simulink model "FK"  (R2024b)
settings: Solver=FixedStepDiscrete  StartTime=0.0  StopTime=Inf  FixedStep=0.001  RelTol=1e-3
model workspace (MAT data in the model file):
  robot : robotics.RigidBodyTree (value not decoded)
values from neighbouring files (symbols this model uses):
  lambda_l_list = [lambda_l_list,se3ToVec(logm(getTransform(robot,q,"l_tcp","l_6")))]    [getDualArmLambdaList.m]
  lambda_rl_list = [lambda_rl_list,se3ToVec(logm(getTransform(robot,q,"l_tcp","l_6")))]    [getDualArmLambdaList.m]
undefined symbols (not defined in the file or in its folder): lambda_r_list
settings Model: Creator=sung  LastModifiedBy=sung
settings HardwareCC: ProdBitPerLong=64  ProdHWDeviceType=Intel->x86-64 (Linux 64)
settings RTWCC: GenCodeOnly=on  Toolchain=CMake

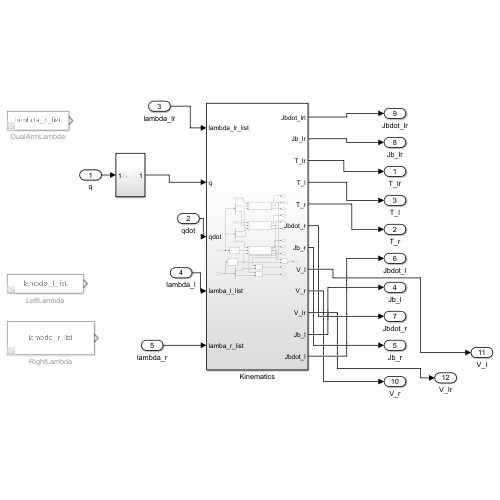
[thumbnail: Simulink's stored preview of the top-level diagram]
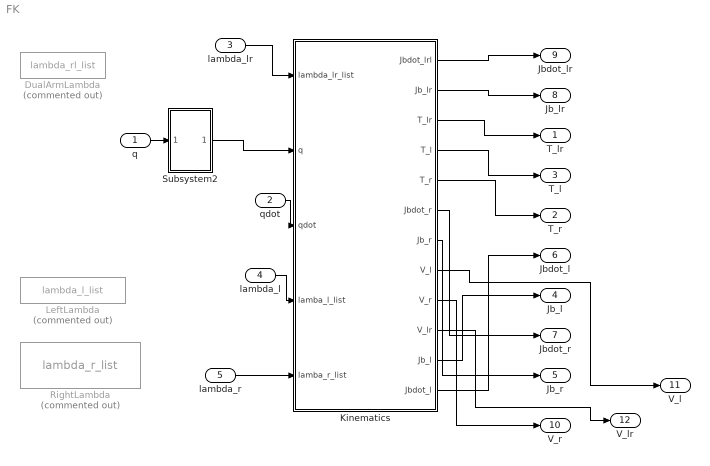
== system FK ==
  q : Inport  PortDimensions=12
  qdot : Inport  Port=2  PortDimensions=12
  lambda_lr : Inport  Port=3  PortDimensions=[6,13]
  lambda_l : Inport  Port=4  PortDimensions=[6,7]
  lambda_r : Inport  Port=5  PortDimensions=[6,7]
  DualArmLambda : Constant  Commented=on  Value=lambda_rl_list
  Kinematics : Subsystem
  LeftLambda : Constant  Commented=on  Value=lambda_l_list
  RightLambda : Constant  Commented=on  Value=lambda_r_list
  Subsystem2 : Subsystem
  T_lr : Outport
  T_r : Outport  Port=2
  T_l : Outport  Port=3
  Jb_l : Outport  Port=4
  Jb_r : Outport  Port=5
  Jbdot_l : Outport  Port=6
  Jbdot_r : Outport  Port=7
  Jb_lr : Outport  Port=8
  Jbdot_lr : Outport  Port=9
  V_r : Outport  Port=10
  V_l : Outport  Port=11
  V_lr : Outport  Port=12
  wires:
  Kinematics/4(T_l) -> T_l/1
  Kinematics/5(T_r) -> T_r/1
  Kinematics/3(T_lr) -> T_lr/1
  Kinematics/2(Jb_lr) -> Jb_lr/1
  Kinematics/1(Jbdot_lrl) -> Jbdot_lr/1
  q/1 -> Subsystem2/1(In1)
  qdot/1 -> Kinematics/3(qdot)
  lambda_lr/1 -> Kinematics/1(lambda_lr_list)
  lambda_l/1 -> Kinematics/4(lamba_l_list)
  lambda_r/1 -> Kinematics/5(lamba_r_list)
  Kinematics/12(Jbdot_l) -> Jbdot_l/1
  Kinematics/11(Jb_l) -> Jb_l/1
  Kinematics/6(Jbdot_r) -> Jbdot_r/1
  Kinematics/7(Jb_r) -> Jb_r/1
  Kinematics/8(V_l) -> V_l/1
  Kinematics/9(V_r) -> V_r/1
  Kinematics/10(V_lr) -> V_lr/1
  Subsystem2/1(Out1) -> Kinematics/2(q)

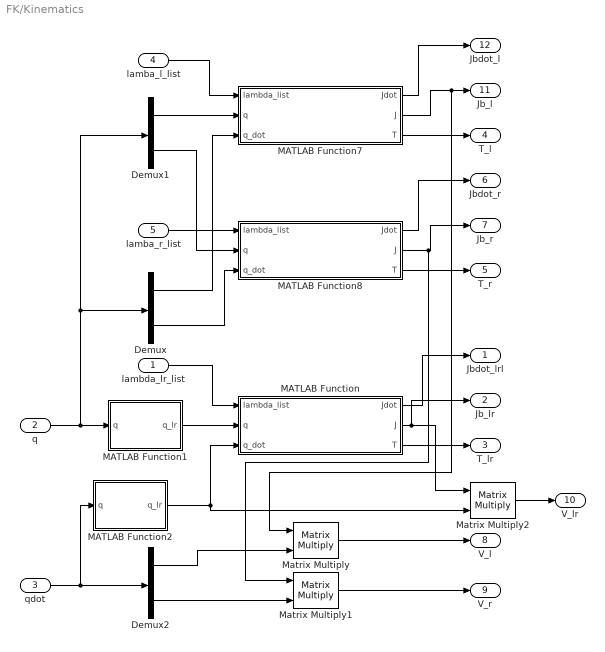
== system FK/Kinematics ==
  lambda_lr_list : Inport
  q : Inport  Port=2
  qdot : Inport  Port=3
  lamba_l_list : Inport  Port=4
  lamba_r_list : Inport  Port=5
  Demux : Demux  Outputs=2
  Demux1 : Demux  Outputs=2
  Demux2 : Demux  Outputs=2
  MATLAB Function : MATLAB Function  TreatAsAtomicUnit=on
  MATLAB Function1 : MATLAB Function  TreatAsAtomicUnit=on
  MATLAB Function2 : MATLAB Function  TreatAsAtomicUnit=on
  MATLAB Function7 : MATLAB Function  TreatAsAtomicUnit=on
  MATLAB Function8 : MATLAB Function  TreatAsAtomicUnit=on
  Matrix Multiply : Product  Multiplication=Matrix(*)
  Matrix Multiply1 : Product  Multiplication=Matrix(*)
  Matrix Multiply2 : Product  Multiplication=Matrix(*)
  Jbdot_lrl : Outport
  Jb_lr : Outport  Port=2
  T_lr : Outport  Port=3
  T_l : Outport  Port=4
  T_r : Outport  Port=5
  Jbdot_r : Outport  Port=6
  Jb_r : Outport  Port=7
  V_l : Outport  Port=8
  V_r : Outport  Port=9
  V_lr : Outport  Port=10
  Jb_l : Outport  Port=11
  Jbdot_l : Outport  Port=12
  wires:
  lamba_l_list/1 -> MATLAB Function7/1(lambda_list)
  MATLAB Function2/1(q_lr) -> Matrix Multiply2/2, MATLAB Function/3(q_dot)
  q/1 -> Demux1/1, Demux/1, MATLAB Function1/1(q)
  Demux/2 -> MATLAB Function8/3(q_dot)
  MATLAB Function/1(Jdot) -> Jbdot_lrl/1
  lamba_r_list/1 -> MATLAB Function8/1(lambda_list)
  Matrix Multiply/1 -> V_l/1
  Demux1/2 -> MATLAB Function8/2(q)
  qdot/1 -> Demux2/1, MATLAB Function2/1(q)
  Demux/1 -> MATLAB Function7/3(q_dot)
  Demux1/1 -> MATLAB Function7/2(q)
  lambda_lr_list/1 -> MATLAB Function/1(lambda_list)
  MATLAB Function1/1(q_lr) -> MATLAB Function/2(q)
  Demux2/1 -> Matrix Multiply/2
  Matrix Multiply1/1 -> V_r/1
  Demux2/2 -> Matrix Multiply1/2
  MATLAB Function7/1(Jdot) -> Jbdot_l/1
  MATLAB Function7/2(J) -> Matrix Multiply/1, Jb_l/1
  MATLAB Function7/3(T) -> T_l/1
  MATLAB Function8/1(Jdot) -> Jbdot_r/1
  MATLAB Function/3(T) -> T_lr/1
  MATLAB Function8/2(J) -> Matrix Multiply1/1, Jb_r/1
  MATLAB Function8/3(T) -> T_r/1
  MATLAB Function/2(J) -> Matrix Multiply2/1, Jb_lr/1
  Matrix Multiply2/1 -> V_lr/1

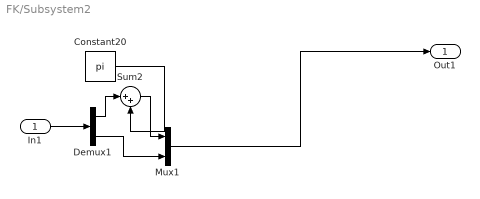
== system FK/Subsystem2 ==
  In1 : Inport
  Constant20 : Constant  Value=pi
  Demux1 : Demux  Outputs=[1,11]
  Mux1 : Mux  Inputs=[1,11]
  Sum2 : Sum  Inputs=|++
  Out1 : Outport
  wires:
  Sum2/1 -> Mux1/1
  Demux1/2 -> Mux1/2
  Constant20/1 -> Sum2/2
  In1/1 -> Demux1/1
  Demux1/1 -> Sum2/1
  Mux1/1 -> Out1/1

== matlab function FK/Kinematics/MATLAB Function1 ==
  data: q input; q_lr output
function q_lr = getQrel(q)
q_lr = zeros(12,1);
q_lr = [-flip(q(1:6));q(7:end)];

== matlab function FK/Kinematics/MATLAB Function ==
  data: Jdot output; J output; lambda_list input; T output; q input; q_dot input
function [Jdot,J,T]=FKJacobian(lambda_list,q,q_dot)
    Ti = eye(4);
    [m,n]=size(lambda_list);
    lamda_z = [0,0,0,0,0,1]';
    ez = [0,0,1]';
    N = length(q);
    J = zeros(6,N);
    Jdot=zeros(6,N);
  
    Ti = exp6(lambda_list(:,end));
    [Ri,pi] = TransToRp(Ti);
    J(:,end)=[Ri'*VecToso3(ez)*pi;Ri'*ez];
    for i =N:-1:1
        Ti = exp6(lambda_list(:,i))*exp6(lamda_z*q(i))*Ti;
 
        [Ri,pi] = TransToRp(Ti);
        if i>1
            J(:,i-1)=[Ri'*VecToso3(ez)*pi;Ri'*ez];
        end

    end
    for i=1:1:N
        Ji = J(:,i);
        dJidt = zeros(6,1);
        for j=1:1:N
            Jj = J(:,j);
            aJiaqj = zeros(6,1);
            if(i<j) 
                aJiaqj = ad(Ji)*Jj;
            end
            dJidt = dJidt+aJiaqj*q_dot(j);
        end
        Jdot(:,i) = dJidt;
    end
    T = Ti;
end

== matlab function FK/Kinematics/MATLAB Function2 ==
  data: q input; q_lr output
function q_lr = getQrel(q)
q_lr = zeros(12,1);
q_lr = [-flip(q(1:6));q(7:end)];

== matlab function FK/Kinematics/MATLAB Function7 ==
  data: Jdot output; J output; lambda_list input; T output; q input; q_dot input
function [Jdot,J,T]=FKJacobian(lambda_list,q,q_dot)
    Ti = eye(4);
    [m,n]=size(lambda_list);
    lamda_z = [0,0,0,0,0,1]';
    ez = [0,0,1]';
    N = length(q);
    J = zeros(6,N);
    Jdot=zeros(6,N);
  
    Ti = exp6(lambda_list(:,end));
    [Ri,pi] = TransToRp(Ti);
    J(:,end)=[Ri'*VecToso3(ez)*pi;Ri'*ez];
    for i =N:-1:1
        Ti = exp6(lambda_list(:,i))*exp6(lamda_z*q(i))*Ti;
 
        [Ri,pi] = TransToRp(Ti);
        if i>1
            J(:,i-1)=[Ri'*VecToso3(ez)*pi;Ri'*ez];
        end

    end
    for i=1:1:N
        Ji = J(:,i);
        dJidt = zeros(6,1);
        for j=1:1:N
            Jj = J(:,j);
            aJiaqj = zeros(6,1);
            if(i<j) 
                aJiaqj = ad(Ji)*Jj;
            end
            dJidt = dJidt+aJiaqj*q_dot(j);
        end
        Jdot(:,i) = dJidt;
    end
    T = Ti;
end

== matlab function FK/Kinematics/MATLAB Function8 ==
  data: Jdot output; J output; lambda_list input; T output; q input; q_dot input
function [Jdot,J,T]=FKJacobian(lambda_list,q,q_dot)
    Ti = eye(4);
    [m,n]=size(lambda_list);
    lamda_z = [0,0,0,0,0,1]';
    ez = [0,0,1]';
    N = length(q);
    J = zeros(6,N);
    Jdot=zeros(6,N);
  
    Ti = exp6(lambda_list(:,end));
    [Ri,pi] = TransToRp(Ti);
    J(:,end)=[Ri'*VecToso3(ez)*pi;Ri'*ez];
    for i =N:-1:1
        Ti = exp6(lambda_list(:,i))*exp6(lamda_z*q(i))*Ti;
 
        [Ri,pi] = TransToRp(Ti);
        if i>1
            J(:,i-1)=[Ri'*VecToso3(ez)*pi;Ri'*ez];
        end

    end
    for i=1:1:N
        Ji = J(:,i);
        dJidt = zeros(6,1);
        for j=1:1:N
            Jj = J(:,j);
            aJiaqj = zeros(6,1);
            if(i<j) 
                aJiaqj = ad(Ji)*Jj;
            end
            dJidt = dJidt+aJiaqj*q_dot(j);
        end
        Jdot(:,i) = dJidt;
    end
    T = Ti;
end
